simulink model "HundredFreqF"  (R2014a)
settings: Solver=ode45  StartTime=0.0  StopTime=10.0  RelTol=1e-3
undefined symbols (not defined in the file): i
libraries: dspsigops x2
settings Model: Creator=Tanvir  LastModifiedBy=Tanvir

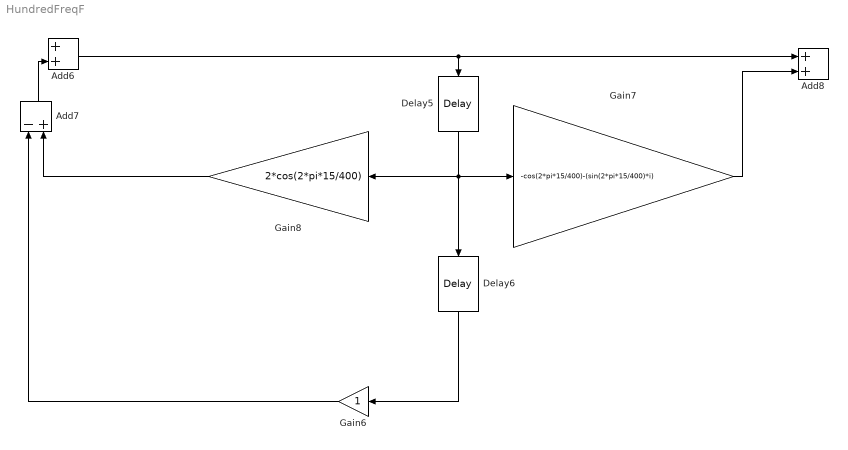
== system HundredFreqF ==
  Add6 : Sum
  Add7 : Sum  Inputs=-+
  Add8 : Sum
  Delay5 : dspsigops/Delay  InputProcessing=Columns as channels (frame based)  dly_unit=Samples  delay=1  ic_detail=off  dif_ic_for_ch=off  dif_ic_for_dly=off  ic=0  reset_popup=None
  Delay6 : dspsigops/Delay  InputProcessing=Columns as channels (frame based)  dly_unit=Samples  delay=1  ic_detail=off  dif_ic_for_ch=off  dif_ic_for_dly=off  ic=0  reset_popup=None
  Gain6 : Gain
  Gain7 : Gain  Gain=-cos(2*pi*15/400)-(sin(2*pi*15/400)*i)
  Gain8 : Gain  Gain=2*cos(2*pi*15/400)
  wires:
  Delay5/1 -> Delay6/1, Gain8/1, Gain7/1
  Delay6/1 -> Gain6/1
  Add6/1 -> Add8/1, Delay5/1
  Gain6/1 -> Add7/1
  Add7/1 -> Add6/2
  Gain7/1 -> Add8/2
  Gain8/1 -> Add7/2
  ? -> Add6/1
